simulink model "sgMdl_IO751_IO752_PROFINETMultiNode"  (R2024b)
settings: Solver=FixedStepAuto  StartTime=0.0  StopTime=inf  RelTol=1e-3  EnableMultiTasking=on
undefined symbols (not defined in the file): C, DiscIntNeverNeededParam, Ts
libraries: slrealtimeutilitieslib x80, speedgoatlib_IO752 x6, speedgoatlib_IO751 x3, simulink x2
(part 1 of 2)
Description:
  | IO751 & IO752 - PROFINET Multi-Node
settings Model: ModifiedByFormat=Speedgoat  Creator=Speedgoat  LastModifiedBy=Speedgoat
settings SolverCC: ConcurrentTasks=on  AlgebraicLoopSolver=TrustRegion  PositivePriorityOrder=on  InsertRTBMode=Never (minimum delay)
settings DataIOCC: SaveFormat=Array  SaveState=on  SignalLoggingName=logsOut
settings OptimizationCC: BlockReduction=off  BooleanDataType=off  OptimizeBlockIOStorage=off  BufferReuse=off  ReuseModelBlockBuffer=off  GlobalBufferReuse=off  ExpressionFolding=off  LocalBlockOutputs=off  InitFltsAndDblsToZero=on  OptimizeDataStoreBuffers=off  BusAssignmentInplaceUpdate=off
settings DebuggingCC: SaveWithParameterizedLinksMsg=none  UnderspecifiedInitializationDetection=Classic  MergeDetectMultiDrivingBlocksExec=none  CheckExecutionContextPreStartOutputMsg=on  SignalResolutionControl=TryResolveAllWithWarning  TasksWithSamePriorityMsg=none  UnconnectedInputMsg=warning  UnconnectedOutputMsg=warning  UnconnectedLineMsg=warning  SFUnexpectedBacktrackingDiag=warning  SFNoUnconditionalDefaultTransitionDiag=warning  SFExecutionAtInitializationDiag=none  ArithmeticOperatorsInVariantConditions=warning
settings HardwareCC: ProdBitPerLong=64  ProdLongLongMode=on  ProdHWDeviceType=Intel->x86-64 (Linux 64)
settings ModelReferenceCC: EnableRefExpFcnMdlSchedulingChecks=on  PropagateSignalLabelsOutOfModel=off
settings SFSimCC: SimUseLocalCustomCode=off  SimTargetLang=C++
settings RTWCC: Description=Speedgoat Real-Time Target Machine  SystemTargetFile=speedgoat.tlc  TemplateMakefile=slrealtime_default_tmf  RTWUseLocalCustomCode=off  Toolchain=Simulink Real-Time Toolchain  BuildConfiguration=Faster Runs  TargetLang=C++  GPUComputeCapability=3.5  DLArmComputeVersion=19.05
settings CodeAppCC: StateflowObjectComments=on
settings SimulinkRealTimeTargetCC: SubcomponentCodeInterfacePackaging=Reusable function  InstructionSetFMA=off  LogToMDFFile=off  SLRTFileLogMaxRuns=10
settings ConfigComp: CovMetricSettings=dw  CovSaveCumulativeToWorkspaceVar=on  CovSaveSingleToWorkspaceVar=on  CovExternalEMLEnable=off  CovSFcnEnable=off  CovBoundaryAbsTol=1.0e-5

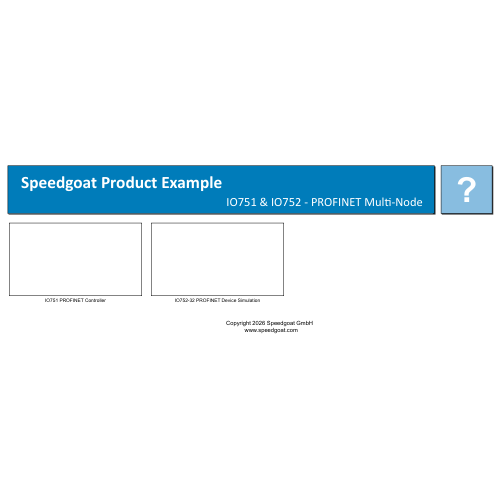
[thumbnail: Simulink's stored preview of the top-level diagram]
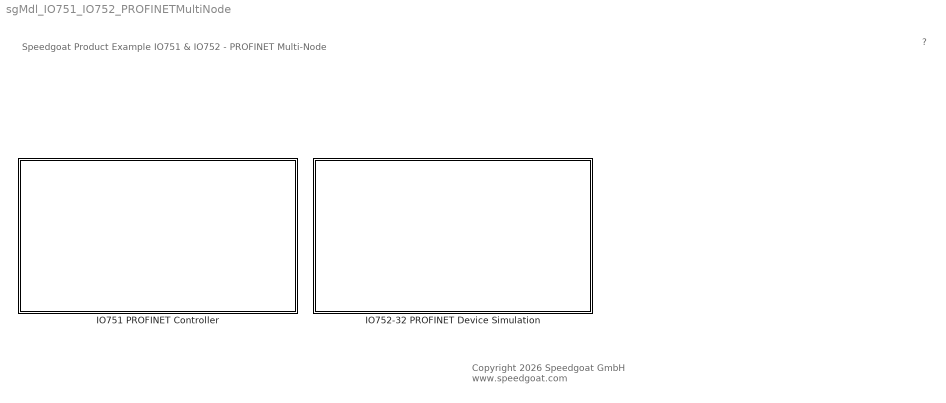
== system sgMdl_IO751_IO752_PROFINETMultiNode ==
  note: Speedgoat Product Example
      | IO751 & IO752 - PROFINET Multi-Node
  note: ?
  note: Copyright 2026 Speedgoat GmbH
      |  www.speedgoat.com
  IO751 PROFINET Controller : Subsystem
  IO752-32 PROFINET Device Simulation : Subsystem

== system sgMdl_IO751_IO752_PROFINETMultiNode/IO751 PROFINET Controller ==
  note: Send
      |
      | Send DO and AO signals to the simulated ET200SP
      | Send control signals and speed setpoints to the simulated SINAMICS drive
  note: Setup
  note: Receive
      |
      | Receive DI and AI signals from the simulated ET200SP
      | Receive status signals and actual speed values from the simulated SINAMICS drive
  "PNM Setup v2 " : speedgoatlib_IO751/PNM Setup v2   id=1  driveLetter=C:  configurationMode=Configuration file  mode=Polling mode  pciSlot=[6,0]  quantityOfAcyclicObjects=0  qtyMods=[1,0,0]  ConfigFile=which('IO751_IO752_MultiNode_m.nxd')  parOptAcyclic=off  protocol=IO751  firmware=PROFINET Controller
      settings: SourceProductName=IO751 PROFINET Controller
  Receive : Subsystem
  Send : Subsystem

== system sgMdl_IO751_IO752_PROFINETMultiNode/IO752-32 PROFINET Device Simulation ==
  Device 1 ET200SP : Subsystem
  Device 2 SINAMICS : Subsystem

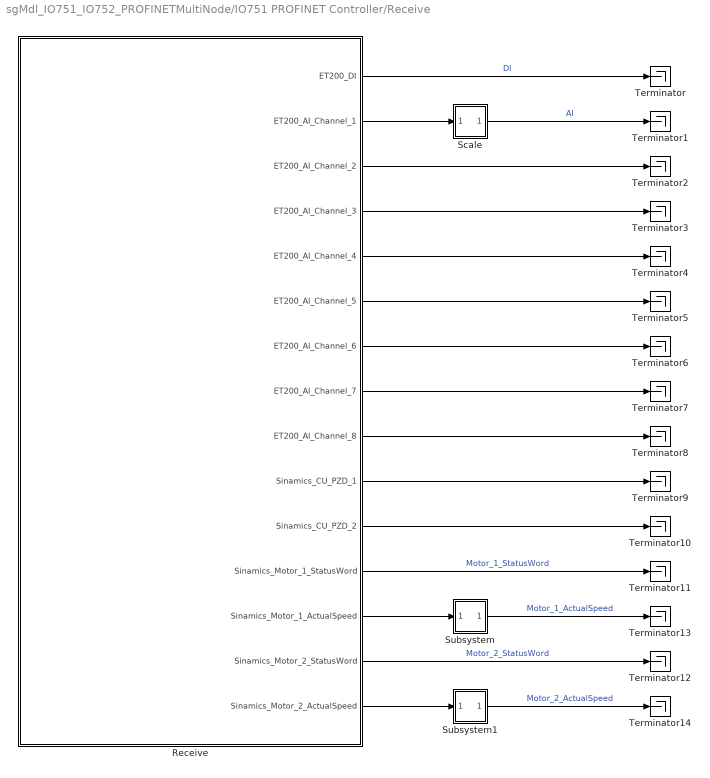
== system sgMdl_IO751_IO752_PROFINETMultiNode/IO751 PROFINET Controller/Receive ==
  Receive : Subsystem
  Scale : Subsystem
  Subsystem : Subsystem
  Subsystem1 : Subsystem
  Terminator{,1..14} (15 alike) : Terminator
  wires:
  Receive/14(Sinamics_Motor_2_StatusWord) -> Terminator12/1  "Motor_2_StatusWord"
  Receive/7(ET200_AI_Channel_6) -> Terminator6/1
  Receive/10(Sinamics_CU_PZD_1) -> Terminator9/1
  Receive/11(Sinamics_CU_PZD_2) -> Terminator10/1
  Receive/8(ET200_AI_Channel_7) -> Terminator7/1
  Receive/2(ET200_AI_Channel_1) -> Scale/1(In1)
  Receive/9(ET200_AI_Channel_8) -> Terminator8/1
  Receive/1(ET200_DI) -> Terminator/1  "DI"
  Receive/4(ET200_AI_Channel_3) -> Terminator3/1
  Receive/12(Sinamics_Motor_1_StatusWord) -> Terminator11/1  "Motor_1_StatusWord"
  Receive/3(ET200_AI_Channel_2) -> Terminator2/1
  Receive/6(ET200_AI_Channel_5) -> Terminator5/1
  Receive/5(ET200_AI_Channel_4) -> Terminator4/1
  Receive/13(Sinamics_Motor_1_ActualSpeed) -> Subsystem/1(In1)
  Subsystem/1(Out1) -> Terminator13/1  "Motor_1_ActualSpeed"
  Receive/15(Sinamics_Motor_2_ActualSpeed) -> Subsystem1/1(In1)
  Subsystem1/1(Out1) -> Terminator14/1  "Motor_2_ActualSpeed"
  Scale/1(Out1) -> Terminator1/1  "AI"

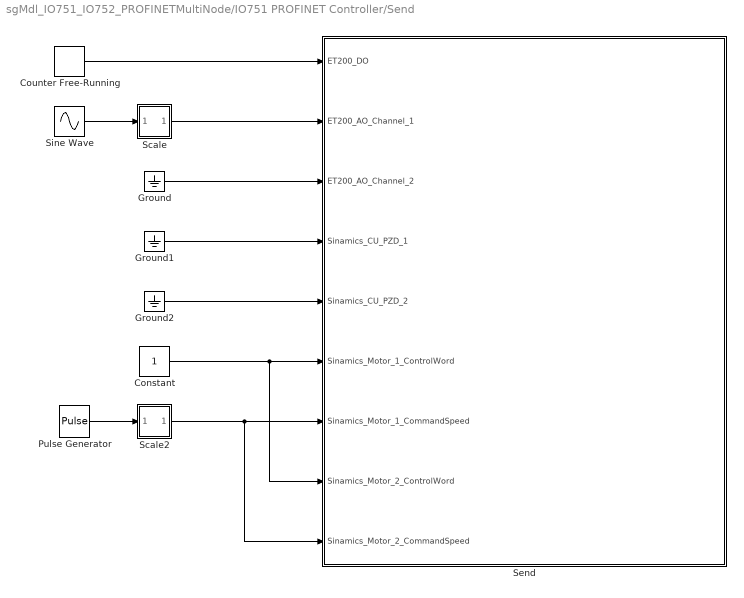
== system sgMdl_IO751_IO752_PROFINETMultiNode/IO751 PROFINET Controller/Send ==
  Constant : Constant  OutDataTypeStr=Inherit: Inherit via back propagation
  Counter Free-Running : simulink/Sources/Counter Free-Running  NumBits=16  tsamp=Ts
  Ground : Ground
  Ground1 : Ground
  Ground2 : Ground
  Pulse Generator : DiscretePulseGenerator  Amplitude=1000  Period=1/Ts*2  PulseWidth=(1/Ts*2)/2  SampleTime=Ts
  Scale : Subsystem
  Scale2 : Subsystem
  Send : Subsystem
  Sine Wave : Sin  SineType=Sample based  Amplitude=10  Frequency=180  Samples=1/Ts*4  SampleTime=Ts
  wires:
  Ground1/1 -> Send/4(Sinamics_CU_PZD_1)
  Ground/1 -> Send/3(ET200_AO_Channel_2)
  Ground2/1 -> Send/5(Sinamics_CU_PZD_2)
  Constant/1 -> Send/8(Sinamics_Motor_2_ControlWord), Send/6(Sinamics_Motor_1_ControlWord)
  Counter Free-Running/1 -> Send/1(ET200_DO)
  Sine Wave/1 -> Scale/1(In1)
  Scale/1(Out1) -> Send/2(ET200_AO_Channel_1)
  Scale2/1(Out1) -> Send/9(Sinamics_Motor_2_CommandSpeed), Send/7(Sinamics_Motor_1_CommandSpeed)
  Pulse Generator/1 -> Scale2/1(In1)

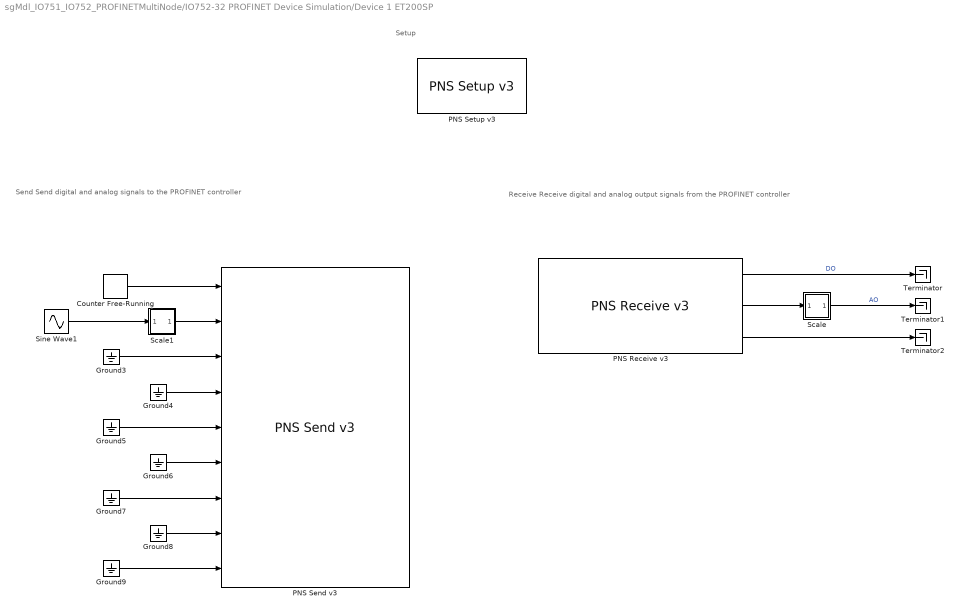
== system sgMdl_IO751_IO752_PROFINETMultiNode/IO752-32 PROFINET Device Simulation/Device 1 ET200SP ==
  note: Receive
      |
      | Receive digital and analog output signals from the PROFINET controller
  note: Setup
  note: Send
      |
      | Send digital and analog signals to the PROFINET controller
  Counter Free-Running : simulink/Sources/Counter Free-Running  NumBits=8  tsamp=Ts
  Ground{3..9} (7 alike) : Ground
  PNS Receive v3 : speedgoatlib_IO752/PNS Receive v3  id=[2 1]  SampleTime=Ts  DataLevel=Data Item  GroupDataItems=off  PortLabel1=off  PortLabel2=on  PortLabel3=off  PnModuleConfig="{ '0', '', 'IM 155-6 PN ST V4.1', '673536', '', '', 'DIM ST V4.1', '', '', '0', '1', ''; '0', '1', '  IM 155-6 PN ST V4.1', '673536', '2', '', 'DIM PN ST V4.1', '1', '', '', '', ''; '0', '32768', '  PN-IO', '673536', '32770', '', 'IDS_1I ST V4.1', '1', '', '', '', ''; '0', '32769', '  Port 1 (2xRJ45)', '673536', '49152', '', 'IDS_1P1 ST RJ45 V3.3', '0', '', '', '', ''; '0', '32770', '  Port 2 (2xRJ45)', '673536', '49152', '', 'IDS_1P2 ST RJ45 V3.3', '0', '', '', '', ''; '1', '', 'DI 8x24VDC ST V1.1', '19787', '', '', 'DI 8x24VDC ST V1.1', '0', '', '', '', ''; '1', '1', '  DI 8x24VDC ST V1.1', '19787', '8', '', 'DI 8x24VDC ST V1.1_01', '1', '{\"Inputs\",[3],[1]}', '', '', ''; '2', '', 'DQ 16x24VDC/0.5A ST V1.1', '19852', '', '', 'DQ 16x24VDC/0,5A ST V1.1', '0', '', '', '', ''; '2', '1', '  DQ 16x24VDC/0.5A ST V1.1', '19852', '16', '', 'DQ 16x24VDC/0,5A ST V1.1_01', '1', '', '{\"Outputs\",[5],[1]}', '', ''; '3', '', 'AI 8xU BA V1.0', '19022', '', '', 'AI 8xU BA', '0', '', '', '', ''; '3', '1', '  AI 8xU BA V1.0', '19022', '8', '', 'AI 8xU BA_01', '1', '{\"I-channel 0\",[4],[1];\"I-channel 1\",[4],[1];\"I-channel 2\",[4],[1];\"I-channel 3\",[4],[1];\"I-channel 4\",[4],[1];\"I-channel 5\",[4],[1];\"I-channel 6\",[4],[1];\"I-channel 7\",[4],[1]}', '', '', ''; '4', '', 'AQ 2xU ST V1.0', '19082', '', '', 'AQ 2xU ST', '0', '', '', '', ''; '4', '1', '  AQ 2xU ST V1.0', '19082', '2', '', 'AQ 2xU ST_01', '1', '', '{\"O-channel 0\",[4],[1];\"O-channel 1\",[4],[1]}', '', '' }"
      settings: SourceProductName=IO752 PROFINET Device
  PNS Send v3 : speedgoatlib_IO752/PNS Send v3  id=[2 1]  SampleTime=Ts  DataLevel=Data Item  GroupDataItems=off  PortLabel1=off  PortLabel2=on  PortLabel3=off  PnModuleConfig="{ '0', '', 'IM 155-6 PN ST V4.1', '673536', '', '', 'DIM ST V4.1', '', '', '0', '1', ''; '0', '1', '  IM 155-6 PN ST V4.1', '673536', '2', '', 'DIM PN ST V4.1', '1', '', '', '', ''; '0', '32768', '  PN-IO', '673536', '32770', '', 'IDS_1I ST V4.1', '1', '', '', '', ''; '0', '32769', '  Port 1 (2xRJ45)', '673536', '49152', '', 'IDS_1P1 ST RJ45 V3.3', '0', '', '', '', ''; '0', '32770', '  Port 2 (2xRJ45)', '673536', '49152', '', 'IDS_1P2 ST RJ45 V3.3', '0', '', '', '', ''; '1', '', 'DI 8x24VDC ST V1.1', '19787', '', '', 'DI 8x24VDC ST V1.1', '0', '', '', '', ''; '1', '1', '  DI 8x24VDC ST V1.1', '19787', '8', '', 'DI 8x24VDC ST V1.1_01', '1', '{\"Inputs\",[3],[1]}', '', '', ''; '2', '', 'DQ 16x24VDC/0.5A ST V1.1', '19852', '', '', 'DQ 16x24VDC/0,5A ST V1.1', '0', '', '', '', ''; '2', '1', '  DQ 16x24VDC/0.5A ST V1.1', '19852', '16', '', 'DQ 16x24VDC/0,5A ST V1.1_01', '1', '', '{\"Outputs\",[5],[1]}', '', ''; '3', '', 'AI 8xU BA V1.0', '19022', '', '', 'AI 8xU BA', '0', '', '', '', ''; '3', '1', '  AI 8xU BA V1.0', '19022', '8', '', 'AI 8xU BA_01', '1', '{\"I-channel 0\",[4],[1];\"I-channel 1\",[4],[1];\"I-channel 2\",[4],[1];\"I-channel 3\",[4],[1];\"I-channel 4\",[4],[1];\"I-channel 5\",[4],[1];\"I-channel 6\",[4],[1];\"I-channel 7\",[4],[1]}', '', '', ''; '4', '', 'AQ 2xU ST V1.0', '19082', '', '', 'AQ 2xU ST', '0', '', '', '', ''; '4', '1', '  AQ 2xU ST V1.0', '19082', '2', '', 'AQ 2xU ST_01', '1', '', '{\"O-channel 0\",[4],[1];\"O-channel 1\",[4],[1]}', '', '' }"
      settings: SourceProductName=IO752 PROFINET Device
  PNS Setup v3 : speedgoatlib_IO752/PNS Setup v3  id=[2 1]  PciSlot=[11,0]  StationName='et200sp'  BusStart=On model start  SystemRedundancy=off  RecordSuccess=on  GsdFile=[pwd, '\IO751_IO752_files\GSDML-V2.33-Siemens-ET200SP-20171124.xml']  VendorId=42  DeviceId=787  OptionalIdentity=off  DeviceType='cifxrepns'  OrderId='1250.1'  HwRev=2  SwRevPrefix='V'  SwRev=[3,0,0]  SerialNumber='0'  ModuleConfigTable="{ '0', '', 'IM 155-6 PN ST V4.1', '673536', '', '', 'DIM ST V4.1', '', '', '0', '1', ''; '0', '1', '  IM 155-6 PN ST V4.1', '673536', '2', '', 'DIM PN ST V4.1', '1', '', '', '', ''; '0', '32768', '  PN-IO', '673536', '32770', '', 'IDS_1I ST V4.1', '1', '', '', '', ''; '0', '32769', '  Port 1 (2xRJ45)', '673536', '49152', '', 'IDS_1P1 ST RJ45 V3.3', '0', '', '', '', ''; '0', '32770', '  Port 2 (2xRJ45)', '673536', '49152', '', 'IDS_1P2 ST RJ45 V3.3', '0', '', '', '', ''; '1', '', 'DI 8x24VDC ST V1.1', '19787', '', '', 'DI 8x24VDC ST V1.1', '0', '', '', '', ''; '1', '1', '  DI 8x24VDC ST V1.1', '19787', '8', '', 'DI 8x24VDC ST V1.1_01', '1', '{\"Inputs\",[3],[1]}', '', '', ''; '2', '', 'DQ 16x24VDC/0.5A ST V1.1', '19852', '', '', 'DQ 16x24VDC/0,5A ST V1.1', '0', '', '', '', ''; '2', '1', '  DQ 16x24VDC/0.5A ST V1.1', '19852', '16', '', 'DQ 16x24VDC/0,5A ST V1.1_01', '1', '', '{\"Outputs\",[5],[1]}', '', ''; '3', '', 'AI 8xU BA V1.0', '19022', '', '', 'AI 8xU BA', '0', '', '', '', ''; '3', '1', '  AI 8xU BA V1.0', '19022', '8', '', 'AI 8xU BA_01', '1', '{\"I-channel 0\",[4],[1];\"I-channel 1\",[4],[1];\"I-channel 2\",[4],[1];\"I-channel 3\",[4],[1];\"I-channel 4\",[4],[1];\"I-channel 5\",[4],[1];\"I-channel 6\",[4],[1];\"I-channel 7\",[4],[1]}', '', '', ''; '4', '', 'AQ 2xU ST V1.0', '19082', '', '', 'AQ 2xU ST', '0', '', '', '', ''; '4', '1', '  AQ 2xU ST V1.0', '19082', '2', '', 'AQ 2xU ST_01', '1', '', '{\"O-channel 0\",[4],[1];\"O-channel 1\",[4],[1]}', '', '' }"
      settings: SourceProductName=IO752 PROFINET Device
  Scale : Subsystem
  Scale1 : Subsystem
  Sine Wave1 : Sin  SineType=Sample based  Amplitude=5  Frequency=180  Samples=1/Ts*4  SampleTime=Ts
  Terminator : Terminator
  Terminator1 : Terminator
  Terminator2 : Terminator
  wires:
  Ground5/1 -> PNS Send v3/5
  PNS Receive v3/3 -> Terminator2/1
  Ground8/1 -> PNS Send v3/8
  Scale/1(Out1) -> Terminator1/1  "AO"
  PNS Receive v3/2 -> Scale/1(In1)
  Ground9/1 -> PNS Send v3/9
  Counter Free-Running/1 -> PNS Send v3/1
  Ground6/1 -> PNS Send v3/6
  Ground3/1 -> PNS Send v3/3
  Sine Wave1/1 -> Scale1/1(In1)
  Ground4/1 -> PNS Send v3/4
  Scale1/1(Out1) -> PNS Send v3/2
  PNS Receive v3/1 -> Terminator/1  "DO"
  Ground7/1 -> PNS Send v3/7

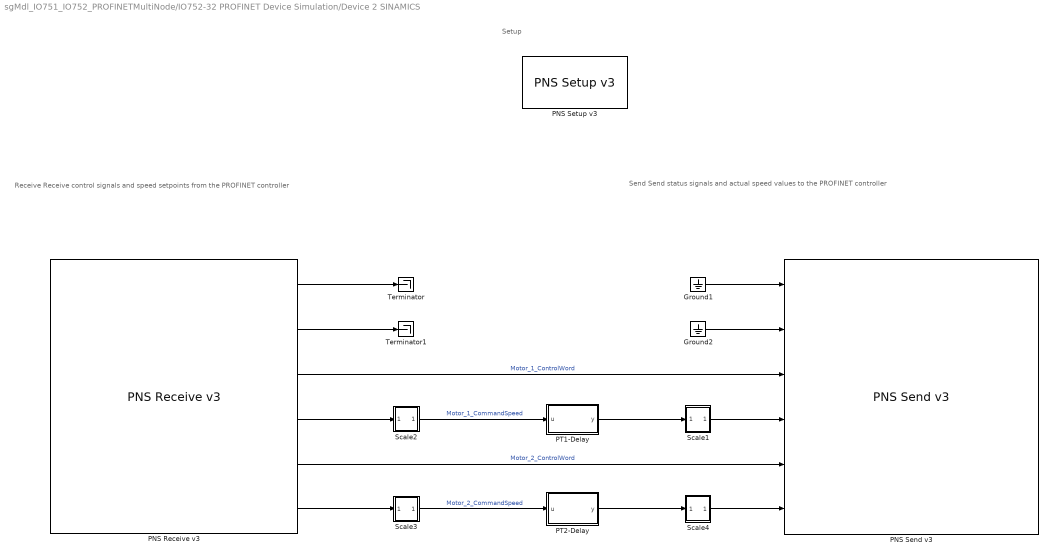
== system sgMdl_IO751_IO752_PROFINETMultiNode/IO752-32 PROFINET Device Simulation/Device 2 SINAMICS ==
  note: Send
      |
      | Send status signals and actual speed values to the PROFINET controller
  note: Setup
  note: Receive
      |
      | Receive control signals and speed setpoints from the PROFINET controller
  Ground1 : Ground
  Ground2 : Ground
  PNS Receive v3 : speedgoatlib_IO752/PNS Receive v3  id=[2 2]  SampleTime=Ts  DataLevel=Data Item  GroupDataItems=off  PortLabel1=on  PortLabel2=on  PortLabel3=off  PnModuleConfig="{ '0', '', 'SINAMICS S120/S150 CU320-2 PN V4.8', '131850', '', '', 'IDD_CU320PN-V4.8', '', '', '0', '0', ''; '0', '1', '  SINAMICS S120/S150 CU320-2 PN V4.8', '131850', '2', '', 'IDS_DAP_CU320PN-V4.8', '1', '', '', '', ''; '0', '32768', '  PN-IO', '131850', '3', '', 'IDS_IF_CU320PN-V4.8', '1', '', '', '', ''; '0', '32769', '  Port 1', '131850', '4', '', 'IDS_P1_CU320PN-V4.8', '1', '', '', '', ''; '0', '32770', '  Port 2', '131850', '5', '', 'IDS_P2_CU320PN-V4.8', '1', '', '', '', ''; '1', '', 'DO Control Unit', '805371922', '', '', 'IDM_CU_45_INT', '0', '', '', '', ''; '1', '1', '  Module Access Point', '805371922', '268500991', '14848', 'IDS_MAP1', '1', '', '', '', ''; '1', '2', '  without PROFIsafe', '805371922', '5001', '14848', 'IDS_NOSAFE', '1', '', '', '', ''; '1', '3', '  SIEMENS telegram 390, PZD-2/2', '805371922', '1342177670', '14848', 'IDS_TEL390_INT2', '0', '{\"Status word or actual value\",[5],[1];\"Status word or actual value\",[5],[1]}', '{\"Control word or setpoint\",[5],[1];\"Control word or setpoint\",[5],[1]}', '', ''; '2', '', 'DO SERVO', '805372083', '', '', 'IDM_SERVO_46_INT', '0', '', '', '', ''; '2', '1', '  Module Access Point', '805372083', '65535', '14848', 'IDS_MAP', '1', '', '', '', ''; '2', '2', '  empty submodule', '805372083', '5000', '14848', 'IDS_EMPTY', '0', '', '', '', ''; '2', '3', '  Standard telegram 1, PZD-2/2', '805372083', '1', '14848', 'IDS_TEL1', '0', '{\"Status word or actual value\",[5],[1];\"Status word or actual value\",[5],[1]}', '{\"Control word or setpoint\",[5],[1];\"Control word or setpoint\",[5],[1]}', '', ''; '3', '', 'DO SERVO', '805372083', '', '', 'IDM_SERVO_46_INT', '0', '', '', '', ''; '3', '1', '  Module Access Point', '805372083', '65535', '14848', 'IDS_MAP', '1', '', '', '', ''; '3', '2', '  empty submodule', '805372083', '5000', '14848', 'IDS_EMPTY', '0', '', '', '', ''; '3', '3', '  Standard telegram 1, PZD-2/2', '805372083', '1', '14848', 'IDS_TEL1', '0', '{\"Status word or actual value\",[5],[1];\"Status word or actual value\",[5],[1]}', '{\"Control word or setpoint\",[5],[1];\"Control word or setpoint\",[5],[1]}', '', '' }"
      settings: SourceProductName=IO752 PROFINET Device
  PNS Send v3 : speedgoatlib_IO752/PNS Send v3  id=[2 2]  SampleTime=Ts  DataLevel=Data Item  GroupDataItems=off  PortLabel1=on  PortLabel2=on  PortLabel3=off  PnModuleConfig="{ '0', '', 'SINAMICS S120/S150 CU320-2 PN V4.8', '131850', '', '', 'IDD_CU320PN-V4.8', '', '', '0', '0', ''; '0', '1', '  SINAMICS S120/S150 CU320-2 PN V4.8', '131850', '2', '', 'IDS_DAP_CU320PN-V4.8', '1', '', '', '', ''; '0', '32768', '  PN-IO', '131850', '3', '', 'IDS_IF_CU320PN-V4.8', '1', '', '', '', ''; '0', '32769', '  Port 1', '131850', '4', '', 'IDS_P1_CU320PN-V4.8', '1', '', '', '', ''; '0', '32770', '  Port 2', '131850', '5', '', 'IDS_P2_CU320PN-V4.8', '1', '', '', '', ''; '1', '', 'DO Control Unit', '805371922', '', '', 'IDM_CU_45_INT', '0', '', '', '', ''; '1', '1', '  Module Access Point', '805371922', '268500991', '14848', 'IDS_MAP1', '1', '', '', '', ''; '1', '2', '  without PROFIsafe', '805371922', '5001', '14848', 'IDS_NOSAFE', '1', '', '', '', ''; '1', '3', '  SIEMENS telegram 390, PZD-2/2', '805371922', '1342177670', '14848', 'IDS_TEL390_INT2', '0', '{\"Status word or actual value\",[5],[1];\"Status word or actual value\",[5],[1]}', '{\"Control word or setpoint\",[5],[1];\"Control word or setpoint\",[5],[1]}', '', ''; '2', '', 'DO SERVO', '805372083', '', '', 'IDM_SERVO_46_INT', '0', '', '', '', ''; '2', '1', '  Module Access Point', '805372083', '65535', '14848', 'IDS_MAP', '1', '', '', '', ''; '2', '2', '  empty submodule', '805372083', '5000', '14848', 'IDS_EMPTY', '0', '', '', '', ''; '2', '3', '  Standard telegram 1, PZD-2/2', '805372083', '1', '14848', 'IDS_TEL1', '0', '{\"Status word or actual value\",[5],[1];\"Status word or actual value\",[5],[1]}', '{\"Control word or setpoint\",[5],[1];\"Control word or setpoint\",[5],[1]}', '', ''; '3', '', 'DO SERVO', '805372083', '', '', 'IDM_SERVO_46_INT', '0', '', '', '', ''; '3', '1', '  Module Access Point', '805372083', '65535', '14848', 'IDS_MAP', '1', '', '', '', ''; '3', '2', '  empty submodule', '805372083', '5000', '14848', 'IDS_EMPTY', '0', '', '', '', ''; '3', '3', '  Standard telegram 1, PZD-2/2', '805372083', '1', '14848', 'IDS_TEL1', '0', '{\"Status word or actual value\",[5],[1];\"Status word or actual value\",[5],[1]}', '{\"Control word or setpoint\",[5],[1];\"Control word or setpoint\",[5],[1]}', '', '' }"
      settings: SourceProductName=IO752 PROFINET Device
  PNS Setup v3 : speedgoatlib_IO752/PNS Setup v3  id=[2 2]  PciSlot=[11,0]  StationName='sinamics-s120-cu320-2pn'  BusStart=On model start  SystemRedundancy=off  RecordSuccess=on  GsdFile=[pwd, '\IO751_IO752_files\GSDML-V2.32-Siemens-Sinamics_S_CU3x0-20160531.xml']  VendorId=42  DeviceId=1281  OptionalIdentity=off  DeviceType='cifxrepns'  OrderId='1250.1'  HwRev=2  SwRevPrefix='V'  SwRev=[3,0,0]  SerialNumber='0'  ModuleConfigTable="{ '0', '', 'SINAMICS S120/S150 CU320-2 PN V4.8', '131850', '', '', 'IDD_CU320PN-V4.8', '', '', '0', '0', ''; '0', '1', '  SINAMICS S120/S150 CU320-2 PN V4.8', '131850', '2', '', 'IDS_DAP_CU320PN-V4.8', '1', '', '', '', ''; '0', '32768', '  PN-IO', '131850', '3', '', 'IDS_IF_CU320PN-V4.8', '1', '', '', '', ''; '0', '32769', '  Port 1', '131850', '4', '', 'IDS_P1_CU320PN-V4.8', '1', '', '', '', ''; '0', '32770', '  Port 2', '131850', '5', '', 'IDS_P2_CU320PN-V4.8', '1', '', '', '', ''; '1', '', 'DO Control Unit', '805371922', '', '', 'IDM_CU_45_INT', '0', '', '', '', ''; '1', '1', '  Module Access Point', '805371922', '268500991', '14848', 'IDS_MAP1', '1', '', '', '', ''; '1', '2', '  without PROFIsafe', '805371922', '5001', '14848', 'IDS_NOSAFE', '1', '', '', '', ''; '1', '3', '  SIEMENS telegram 390, PZD-2/2', '805371922', '1342177670', '14848', 'IDS_TEL390_INT2', '0', '{\"Status word or actual value\",[5],[1];\"Status word or actual value\",[5],[1]}', '{\"Control word or setpoint\",[5],[1];\"Control word or setpoint\",[5],[1]}', '', ''; '2', '', 'DO SERVO', '805372083', '', '', 'IDM_SERVO_46_INT', '0', '', '', '', ''; '2', '1', '  Module Access Point', '805372083', '65535', '14848', 'IDS_MAP', '1', '', '', '', ''; '2', '2', '  empty submodule', '805372083', '5000', '14848', 'IDS_EMPTY', '0', '', '', '', ''; '2', '3', '  Standard telegram 1, PZD-2/2', '805372083', '1', '14848', 'IDS_TEL1', '0', '{\"Status word or actual value\",[5],[1];\"Status word or actual value\",[5],[1]}', '{\"Control word or setpoint\",[5],[1];\"Control word or setpoint\",[5],[1]}', '', ''; '3', '', 'DO SERVO', '805372083', '', '', 'IDM_SERVO_46_INT', '0', '', '', '', ''; '3', '1', '  Module Access Point', '805372083', '65535', '14848', 'IDS_MAP', '1', '', '', '', ''; '3', '2', '  empty submodule', '805372083', '5000', '14848', 'IDS_EMPTY', '0', '', '', '', ''; '3', '3', '  Standard telegram 1, PZD-2/2', '805372083', '1', '14848', 'IDS_TEL1', '0', '{\"Status word or actual value\",[5],[1];\"Status word or actual value\",[5],[1]}', '{\"Control word or setpoint\",[5],[1];\"Control word or setpoint\",[5],[1]}', '', '' }"
      settings: SourceProductName=IO752 PROFINET Device
  PT1-Delay : Subsystem
  PT2-Delay : Subsystem
  Scale1 : Subsystem
  Scale2 : Subsystem
  Scale3 : Subsystem
  Scale4 : Subsystem
  Terminator : Terminator
  Terminator1 : Terminator
  wires:
  PNS Receive v3/1 -> Terminator/1
  PNS Receive v3/2 -> Terminator1/1
  PNS Receive v3/4 -> Scale2/1(In1)
  PNS Receive v3/6 -> Scale3/1(In1)
  Scale3/1(Out1) -> PT2-Delay/1(u)  "Motor_2_CommandSpeed"
  PT2-Delay/1(y) -> Scale4/1(In2)
  PT1-Delay/1(y) -> Scale1/1(In2)
  Scale2/1(Out1) -> PT1-Delay/1(u)  "Motor_1_CommandSpeed"
  Scale1/1(Out1) -> PNS Send v3/4
  Scale4/1(Out1) -> PNS Send v3/6
  PNS Receive v3/5 -> PNS Send v3/5  "Motor_2_ControlWord"
  PNS Receive v3/3 -> PNS Send v3/3  "Motor_1_ControlWord"
  Ground1/1 -> PNS Send v3/1
  Ground2/1 -> PNS Send v3/2

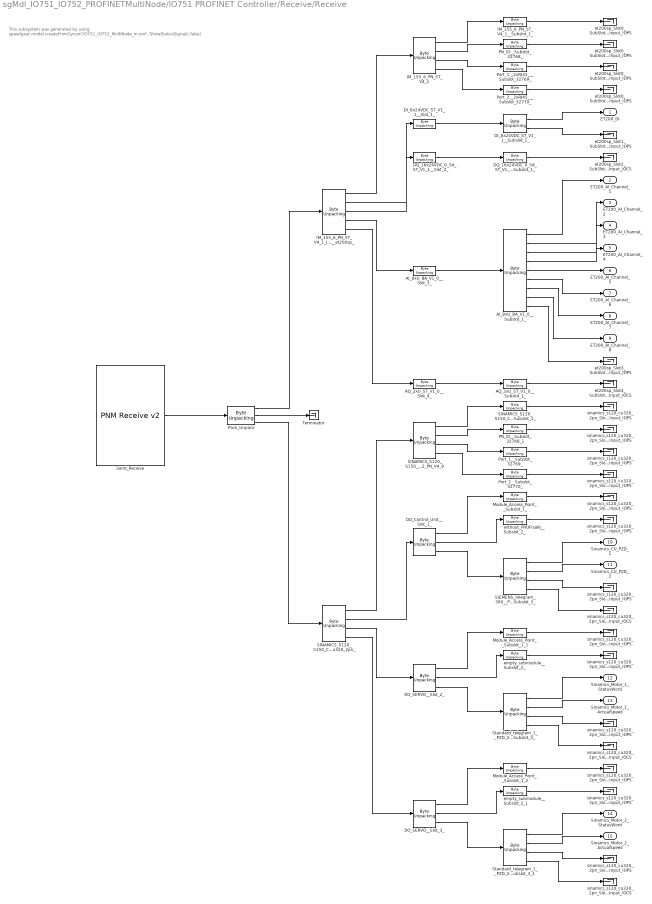
== system sgMdl_IO751_IO752_PROFINETMultiNode/IO751 PROFINET Controller/Receive/Receive ==
  note: This subsystem was generated by using speedgoat.model.createFromSycon('IO751_IO752_MultiNode_m.xml','ShowStatusSignals',false)
  AI_8xU_BA_V1_0__Slot_3_ : slrealtimeutilitieslib/Byte Unpacking  MaskUnpackedDataTypes={'uint8'}  MaskUnpackedDataSizes={[17]}  MaskAlignment=1
  AI_8xU_BA_V1_0__Subslot_1_ : slrealtimeutilitieslib/Byte Unpacking  MaskUnpackedDataTypes={'int16','int16','int16','int16','int16','int16','int16','int16','uint8'}  MaskUnpackedDataSizes={[1],[1],[1],[1],[1],[1],[1],[1],[1]}  MaskAlignment=1
  AQ_2xU_ST_V1_0__Slot_4_ : slrealtimeutilitieslib/Byte Unpacking  MaskUnpackedDataTypes={'uint8'}  MaskUnpackedDataSizes={[1]}  MaskAlignment=1
  AQ_2xU_ST_V1_0__Subslot_1_ : slrealtimeutilitieslib/Byte Unpacking  MaskUnpackedDataTypes={'uint8'}  MaskUnpackedDataSizes={[1]}  MaskAlignment=1
  DI_8x24VDC_ST_V1_1__Slot_1_ : slrealtimeutilitieslib/Byte Unpacking  MaskUnpackedDataTypes={'uint8'}  MaskUnpackedDataSizes={[2]}  MaskAlignment=1
  DI_8x24VDC_ST_V1_1__Subslot_1_ : slrealtimeutilitieslib/Byte Unpacking  MaskUnpackedDataTypes={'uint8','uint8'}  MaskUnpackedDataSizes={[1],[1]}  MaskAlignment=1
  DO_Control_Unit__Slot_1_ : slrealtimeutilitieslib/Byte Unpacking  MaskUnpackedDataTypes={'uint8','uint8','uint8'}  MaskUnpackedDataSizes={[1],[1],[6]}  MaskAlignment=1
  DO_SERVO__Slot_2_ : slrealtimeutilitieslib/Byte Unpacking  MaskUnpackedDataTypes={'uint8','uint8','uint8'}  MaskUnpackedDataSizes={[1],[1],[6]}  MaskAlignment=1
  DO_SERVO__Slot_3_ : slrealtimeutilitieslib/Byte Unpacking  MaskUnpackedDataTypes={'uint8','uint8','uint8'}  MaskUnpackedDataSizes={[1],[1],[6]}  MaskAlignment=1
  DQ_16x24VDC_0_5A_ST_V1_1__Slot_2_ : slrealtimeutilitieslib/Byte Unpacking  MaskUnpackedDataTypes={'uint8'}  MaskUnpackedDataSizes={[1]}  MaskAlignment=1
  DQ_16x24VDC_0_5A_ST_V1_1__Subslot_1_ : slrealtimeutilitieslib/Byte Unpacking  MaskUnpackedDataTypes={'uint8'}  MaskUnpackedDataSizes={[1]}  MaskAlignment=1
  IM_155_6_PN_ST_V4_1 : slrealtimeutilitieslib/Byte Unpacking  MaskUnpackedDataTypes={'uint8','uint8','uint8','uint8'}  MaskUnpackedDataSizes={[1],[1],[1],[1]}  MaskAlignment=1
  IM_155_6_PN_ST_V4_1_IM_155_6_PN_ST_V4_1__et200sp_ : slrealtimeutilitieslib/Byte Unpacking  MaskUnpackedDataTypes={'uint8','uint8','uint8','uint8','uint8'}  MaskUnpackedDataSizes={[4],[2],[1],[17],[1]}  MaskAlignment=1
  IM_155_6_PN_ST_V4_1__Subslot_1_ : slrealtimeutilitieslib/Byte Unpacking  MaskUnpackedDataTypes={'uint8'}  MaskUnpackedDataSizes={[1]}  MaskAlignment=1
  Module_Access_Point__Subslot_1_ : slrealtimeutilitieslib/Byte Unpacking  MaskUnpackedDataTypes={'uint8'}  MaskUnpackedDataSizes={[1]}  MaskAlignment=1
  Module_Access_Point__Subslot_1_1 : slrealtimeutilitieslib/Byte Unpacking  MaskUnpackedDataTypes={'uint8'}  MaskUnpackedDataSizes={[1]}  MaskAlignment=1
  Module_Access_Point__Subslot_1_2 : slrealtimeutilitieslib/Byte Unpacking  MaskUnpackedDataTypes={'uint8'}  MaskUnpackedDataSizes={[1]}  MaskAlignment=1
  PN_IO__Subslot_32768_ : slrealtimeutilitieslib/Byte Unpacking  MaskUnpackedDataTypes={'uint8'}  MaskUnpackedDataSizes={[1]}  MaskAlignment=1
  PN_IO__Subslot_32768_1 : slrealtimeutilitieslib/Byte Unpacking  MaskUnpackedDataTypes={'uint8'}  MaskUnpackedDataSizes={[1]}  MaskAlignment=1
  Pack_Unpack : slrealtimeutilitieslib/Byte Unpacking  MaskUnpackedDataTypes={'uint8','uint8','uint8'}  MaskUnpackedDataSizes={[25],[3],[28]}  MaskAlignment=1
  Port_1__2xRJ45___Subslot_32769_ : slrealtimeutilitieslib/Byte Unpacking  MaskUnpackedDataTypes={'uint8'}  MaskUnpackedDataSizes={[1]}  MaskAlignment=1
  Port_1__Subslot_32769_ : slrealtimeutilitieslib/Byte Unpacking  MaskUnpackedDataTypes={'uint8'}  MaskUnpackedDataSizes={[1]}  MaskAlignment=1
  Port_2__2xRJ45___Subslot_32770_ : slrealtimeutilitieslib/Byte Unpacking  MaskUnpackedDataTypes={'uint8'}  MaskUnpackedDataSizes={[1]}  MaskAlignment=1
  Port_2__Subslot_32770_ : slrealtimeutilitieslib/Byte Unpacking  MaskUnpackedDataTypes={'uint8'}  MaskUnpackedDataSizes={[1]}  MaskAlignment=1
  SIEMENS_telegram_390__PZD_2_2__Subslot_3_ : slrealtimeutilitieslib/Byte Unpacking  MaskUnpackedDataTypes={'uint16','uint16','uint8','uint8'}  MaskUnpackedDataSizes={[1],[1],[1],[1]}  MaskAlignment=1
  SINAMICS_S120_S150_CU320_2_PN_V4_8 : slrealtimeutilitieslib/Byte Unpacking  MaskUnpackedDataTypes={'uint8','uint8','uint8','uint8'}  MaskUnpackedDataSizes={[1],[1],[1],[1]}  MaskAlignment=1
  SINAMICS_S120_S150_CU320_2_PN_V4_8_SINAMICS_S120_S150_CU320_2_PN_V4_8__sinamics_s120_cu320_2pn_ : slrealtimeutilitieslib/Byte Unpacking  MaskUnpackedDataTypes={'uint8','uint8','uint8','uint8'}  MaskUnpackedDataSizes={[4],[8],[8],[8]}  MaskAlignment=1
  SINAMICS_S120_S150_CU320_2_PN_V4_8__Subslot_1_ : slrealtimeutilitieslib/Byte Unpacking  MaskUnpackedDataTypes={'uint8'}  MaskUnpackedDataSizes={[1]}  MaskAlignment=1
  Send_Receive : speedgoatlib_IO751/PNM Receive v2   id=1  portType=1 port with n element vector of type UINT8  inputOutput=56  sampleTime=Ts
      settings: SourceProductName=IO751 PROFINET Controller
  Standard_telegram_1__PZD_2_2__Subslot_3_ : slrealtimeutilitieslib/Byte Unpacking  MaskUnpackedDataTypes={'uint16','int16','uint8','uint8'}  MaskUnpackedDataSizes={[1],[1],[1],[1]}  MaskAlignment=1
  Standard_telegram_1__PZD_2_2__Subslot_3_1 : slrealtimeutilitieslib/Byte Unpacking  MaskUnpackedDataTypes={'uint16','int16','uint8','uint8'}  MaskUnpackedDataSizes={[1],[1],[1],[1]}  MaskAlignment=1
  Terminator : Terminator
  empty_submodule__Subslot_2_ : slrealtimeutilitieslib/Byte Unpacking  MaskUnpackedDataTypes={'uint8'}  MaskUnpackedDataSizes={[1]}  MaskAlignment=1
  empty_submodule__Subslot_2_1 : slrealtimeutilitieslib/Byte Unpacking  MaskUnpackedDataTypes={'uint8'}  MaskUnpackedDataSizes={[1]}  MaskAlignment=1
  et200sp_Slot0_SubSlot1_Input_IOPS : Terminator
  et200sp_Slot0_SubSlot32768_Input_IOPS : Terminator
  et200sp_Slot0_SubSlot32769_Input_IOPS : Terminator
  et200sp_Slot0_SubSlot32770_Input_IOPS : Terminator
  et200sp_Slot1_SubSlot1_Input_IOPS : Terminator
  et200sp_Slot2_SubSlot1_Input_IOCS : Terminator
  et200sp_Slot3_SubSlot1_Input_IOPS : Terminator
  et200sp_Slot4_SubSlot1_Input_IOCS : Terminator
  sinamics_s120_cu320_2pn_Slot0_SubSlot1_Input_IOPS : Terminator
  sinamics_s120_cu320_2pn_Slot0_SubSlot32768_Input_IOPS : Terminator
  sinamics_s120_cu320_2pn_Slot0_SubSlot32769_Input_IOPS : Terminator
  sinamics_s120_cu320_2pn_Slot0_SubSlot32770_Input_IOPS : Terminator
  sinamics_s120_cu320_2pn_Slot1_SubSlot1_Input_IOPS : Terminator
  sinamics_s120_cu320_2pn_Slot1_SubSlot2_Input_IOPS : Terminator
  sinamics_s120_cu320_2pn_Slot1_SubSlot3_Input_IOCS : Terminator
  sinamics_s120_cu320_2pn_Slot1_SubSlot3_Input_IOPS : Terminator
  sinamics_s120_cu320_2pn_Slot2_SubSlot1_Input_IOPS : Terminator
  sinamics_s120_cu320_2pn_Slot2_SubSlot2_Input_IOPS : Terminator
  sinamics_s120_cu320_2pn_Slot2_SubSlot3_Input_IOCS : Terminator
  sinamics_s120_cu320_2pn_Slot2_SubSlot3_Input_IOPS : Terminator
  sinamics_s120_cu320_2pn_Slot3_SubSlot1_Input_IOPS : Terminator
  sinamics_s120_cu320_2pn_Slot3_SubSlot2_Input_IOPS : Terminator
  sinamics_s120_cu320_2pn_Slot3_SubSlot3_Input_IOCS : Terminator
  sinamics_s120_cu320_2pn_Slot3_SubSlot3_Input_IOPS : Terminator
  without_PROFIsafe__Subslot_2_ : slrealtimeutilitieslib/Byte Unpacking  MaskUnpackedDataTypes={'uint8'}  MaskUnpackedDataSizes={[1]}  MaskAlignment=1
  ET200_DI : Outport  OutDataTypeStr=uint8  PortDimensions=1
  ET200_AI_Channel_1 : Outport  Port=2  OutDataTypeStr=int16  PortDimensions=1
  ET200_AI_Channel_2 : Outport  Port=3  OutDataTypeStr=int16  PortDimensions=1
  ET200_AI_Channel_3 : Outport  Port=4  OutDataTypeStr=int16  PortDimensions=1
  ET200_AI_Channel_4 : Outport  Port=5  OutDataTypeStr=int16  PortDimensions=1
  ET200_AI_Channel_5 : Outport  Port=6  OutDataTypeStr=int16  PortDimensions=1
  ET200_AI_Channel_6 : Outport  Port=7  OutDataTypeStr=int16  PortDimensions=1
  ET200_AI_Channel_7 : Outport  Port=8  OutDataTypeStr=int16  PortDimensions=1
  ET200_AI_Channel_8 : Outport  Port=9  OutDataTypeStr=int16  PortDimensions=1
  Sinamics_CU_PZD_1 : Outport  Port=10  OutDataTypeStr=uint16  PortDimensions=1
  Sinamics_CU_PZD_2 : Outport  Port=11  OutDataTypeStr=uint16  PortDimensions=1
  Sinamics_Motor_1_StatusWord : Outport  Port=12  OutDataTypeStr=uint16  PortDimensions=1
  Sinamics_Motor_1_ActualSpeed : Outport  Port=13  OutDataTypeStr=int16  PortDimensions=1
  Sinamics_Motor_2_StatusWord : Outport  Port=14  OutDataTypeStr=uint16  PortDimensions=1
  Sinamics_Motor_2_ActualSpeed : Outport  Port=15  OutDataTypeStr=int16  PortDimensions=1
  wires:
  IM_155_6_PN_ST_V4_1__Subslot_1_/1 -> et200sp_Slot0_SubSlot1_Input_IOPS/1
  PN_IO__Subslot_32768_/1 -> et200sp_Slot0_SubSlot32768_Input_IOPS/1
  Port_1__2xRJ45___Subslot_32769_/1 -> et200sp_Slot0_SubSlot32769_Input_IOPS/1
  Port_2__2xRJ45___Subslot_32770_/1 -> et200sp_Slot0_SubSlot32770_Input_IOPS/1
  IM_155_6_PN_ST_V4_1/1 -> IM_155_6_PN_ST_V4_1__Subslot_1_/1
  IM_155_6_PN_ST_V4_1/2 -> PN_IO__Subslot_32768_/1
  IM_155_6_PN_ST_V4_1/3 -> Port_1__2xRJ45___Subslot_32769_/1
  IM_155_6_PN_ST_V4_1/4 -> Port_2__2xRJ45___Subslot_32770_/1
  DI_8x24VDC_ST_V1_1__Subslot_1_/1 -> ET200_DI/1
  DI_8x24VDC_ST_V1_1__Subslot_1_/2 -> et200sp_Slot1_SubSlot1_Input_IOPS/1
  DI_8x24VDC_ST_V1_1__Slot_1_/1 -> DI_8x24VDC_ST_V1_1__Subslot_1_/1
  DQ_16x24VDC_0_5A_ST_V1_1__Subslot_1_/1 -> et200sp_Slot2_SubSlot1_Input_IOCS/1
  DQ_16x24VDC_0_5A_ST_V1_1__Slot_2_/1 -> DQ_16x24VDC_0_5A_ST_V1_1__Subslot_1_/1
  AI_8xU_BA_V1_0__Subslot_1_/1 -> ET200_AI_Channel_1/1
  AI_8xU_BA_V1_0__Subslot_1_/2 -> ET200_AI_Channel_2/1
  AI_8xU_BA_V1_0__Subslot_1_/3 -> ET200_AI_Channel_3/1
  AI_8xU_BA_V1_0__Subslot_1_/4 -> ET200_AI_Channel_4/1
  AI_8xU_BA_V1_0__Subslot_1_/5 -> ET200_AI_Channel_5/1
  AI_8xU_BA_V1_0__Subslot_1_/6 -> ET200_AI_Channel_6/1
  AI_8xU_BA_V1_0__Subslot_1_/7 -> ET200_AI_Channel_7/1
  AI_8xU_BA_V1_0__Subslot_1_/8 -> ET200_AI_Channel_8/1
  AI_8xU_BA_V1_0__Subslot_1_/9 -> et200sp_Slot3_SubSlot1_Input_IOPS/1
  AI_8xU_BA_V1_0__Slot_3_/1 -> AI_8xU_BA_V1_0__Subslot_1_/1
  AQ_2xU_ST_V1_0__Subslot_1_/1 -> et200sp_Slot4_SubSlot1_Input_IOCS/1
  AQ_2xU_ST_V1_0__Slot_4_/1 -> AQ_2xU_ST_V1_0__Subslot_1_/1
  IM_155_6_PN_ST_V4_1_IM_155_6_PN_ST_V4_1__et200sp_/1 -> IM_155_6_PN_ST_V4_1/1
  IM_155_6_PN_ST_V4_1_IM_155_6_PN_ST_V4_1__et200sp_/2 -> DI_8x24VDC_ST_V1_1__Slot_1_/1
  IM_155_6_PN_ST_V4_1_IM_155_6_PN_ST_V4_1__et200sp_/3 -> DQ_16x24VDC_0_5A_ST_V1_1__Slot_2_/1
  IM_155_6_PN_ST_V4_1_IM_155_6_PN_ST_V4_1__et200sp_/4 -> AI_8xU_BA_V1_0__Slot_3_/1
  IM_155_6_PN_ST_V4_1_IM_155_6_PN_ST_V4_1__et200sp_/5 -> AQ_2xU_ST_V1_0__Slot_4_/1
  SINAMICS_S120_S150_CU320_2_PN_V4_8__Subslot_1_/1 -> sinamics_s120_cu320_2pn_Slot0_SubSlot1_Input_IOPS/1
  PN_IO__Subslot_32768_1/1 -> sinamics_s120_cu320_2pn_Slot0_SubSlot32768_Input_IOPS/1
  Port_1__Subslot_32769_/1 -> sinamics_s120_cu320_2pn_Slot0_SubSlot32769_Input_IOPS/1
  Port_2__Subslot_32770_/1 -> sinamics_s120_cu320_2pn_Slot0_SubSlot32770_Input_IOPS/1
  SINAMICS_S120_S150_CU320_2_PN_V4_8/1 -> SINAMICS_S120_S150_CU320_2_PN_V4_8__Subslot_1_/1
  SINAMICS_S120_S150_CU320_2_PN_V4_8/2 -> PN_IO__Subslot_32768_1/1
  SINAMICS_S120_S150_CU320_2_PN_V4_8/3 -> Port_1__Subslot_32769_/1
  SINAMICS_S120_S150_CU320_2_PN_V4_8/4 -> Port_2__Subslot_32770_/1
  Module_Access_Point__Subslot_1_/1 -> sinamics_s120_cu320_2pn_Slot1_SubSlot1_Input_IOPS/1
  without_PROFIsafe__Subslot_2_/1 -> sinamics_s120_cu320_2pn_Slot1_SubSlot2_Input_IOPS/1
  SIEMENS_telegram_390__PZD_2_2__Subslot_3_/1 -> Sinamics_CU_PZD_1/1
  SIEMENS_telegram_390__PZD_2_2__Subslot_3_/2 -> Sinamics_CU_PZD_2/1
  SIEMENS_telegram_390__PZD_2_2__Subslot_3_/3 -> sinamics_s120_cu320_2pn_Slot1_SubSlot3_Input_IOPS/1
  SIEMENS_telegram_390__PZD_2_2__Subslot_3_/4 -> sinamics_s120_cu320_2pn_Slot1_SubSlot3_Input_IOCS/1
  DO_Control_Unit__Slot_1_/1 -> Module_Access_Point__Subslot_1_/1
  DO_Control_Unit__Slot_1_/2 -> without_PROFIsafe__Subslot_2_/1
  DO_Control_Unit__Slot_1_/3 -> SIEMENS_telegram_390__PZD_2_2__Subslot_3_/1
  Module_Access_Point__Subslot_1_1/1 -> sinamics_s120_cu320_2pn_Slot2_SubSlot1_Input_IOPS/1
  empty_submodule__Subslot_2_/1 -> sinamics_s120_cu320_2pn_Slot2_SubSlot2_Input_IOPS/1
  Standard_telegram_1__PZD_2_2__Subslot_3_/1 -> Sinamics_Motor_1_StatusWord/1
  Standard_telegram_1__PZD_2_2__Subslot_3_/2 -> Sinamics_Motor_1_ActualSpeed/1
  Standard_telegram_1__PZD_2_2__Subslot_3_/3 -> sinamics_s120_cu320_2pn_Slot2_SubSlot3_Input_IOPS/1
  Standard_telegram_1__PZD_2_2__Subslot_3_/4 -> sinamics_s120_cu320_2pn_Slot2_SubSlot3_Input_IOCS/1
  DO_SERVO__Slot_2_/1 -> Module_Access_Point__Subslot_1_1/1
  DO_SERVO__Slot_2_/2 -> empty_submodule__Subslot_2_/1
  DO_SERVO__Slot_2_/3 -> Standard_telegram_1__PZD_2_2__Subslot_3_/1
  Module_Access_Point__Subslot_1_2/1 -> sinamics_s120_cu320_2pn_Slot3_SubSlot1_Input_IOPS/1
  empty_submodule__Subslot_2_1/1 -> sinamics_s120_cu320_2pn_Slot3_SubSlot2_Input_IOPS/1
  Standard_telegram_1__PZD_2_2__Subslot_3_1/1 -> Sinamics_Motor_2_StatusWord/1
  Standard_telegram_1__PZD_2_2__Subslot_3_1/2 -> Sinamics_Motor_2_ActualSpeed/1
  Standard_telegram_1__PZD_2_2__Subslot_3_1/3 -> sinamics_s120_cu320_2pn_Slot3_SubSlot3_Input_IOPS/1
  Standard_telegram_1__PZD_2_2__Subslot_3_1/4 -> sinamics_s120_cu320_2pn_Slot3_SubSlot3_Input_IOCS/1
  DO_SERVO__Slot_3_/1 -> Module_Access_Point__Subslot_1_2/1
  DO_SERVO__Slot_3_/2 -> empty_submodule__Subslot_2_1/1
  DO_SERVO__Slot_3_/3 -> Standard_telegram_1__PZD_2_2__Subslot_3_1/1
  SINAMICS_S120_S150_CU320_2_PN_V4_8_SINAMICS_S120_S150_CU320_2_PN_V4_8__sinamics_s120_cu320_2pn_/1 -> SINAMICS_S120_S150_CU320_2_PN_V4_8/1
  SINAMICS_S120_S150_CU320_2_PN_V4_8_SINAMICS_S120_S150_CU320_2_PN_V4_8__sinamics_s120_cu320_2pn_/2 -> DO_Control_Unit__Slot_1_/1
  SINAMICS_S120_S150_CU320_2_PN_V4_8_SINAMICS_S120_S150_CU320_2_PN_V4_8__sinamics_s120_cu320_2pn_/3 -> DO_SERVO__Slot_2_/1
  SINAMICS_S120_S150_CU320_2_PN_V4_8_SINAMICS_S120_S150_CU320_2_PN_V4_8__sinamics_s120_cu320_2pn_/4 -> DO_SERVO__Slot_3_/1
  Pack_Unpack/1 -> IM_155_6_PN_ST_V4_1_IM_155_6_PN_ST_V4_1__et200sp_/1
  Send_Receive/1 -> Pack_Unpack/1
  Pack_Unpack/3 -> SINAMICS_S120_S150_CU320_2_PN_V4_8_SINAMICS_S120_S150_CU320_2_PN_V4_8__sinamics_s120_cu320_2pn_/1
  Pack_Unpack/2 -> Terminator/1

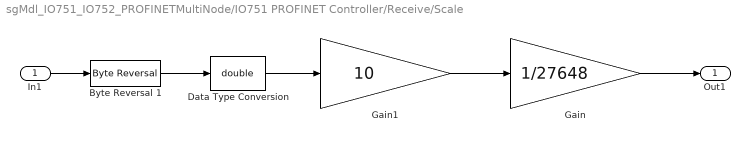
== system sgMdl_IO751_IO752_PROFINETMultiNode/IO751 PROFINET Controller/Receive/Scale ==
  In1 : Inport
  Byte Reversal 1 : slrealtimeutilitieslib/Byte Reversal  numInp=1
  Data Type Conversion : DataTypeConversion  OutDataTypeStr=double  SaturateOnIntegerOverflow=off  RndMeth=Floor
  Gain : Gain  Gain=1/27648
  Gain1 : Gain  Gain=10
  Out1 : Outport
  wires:
  Gain/1 -> Out1/1
  In1/1 -> Byte Reversal 1/1
  Byte Reversal 1/1 -> Data Type Conversion/1
  Data Type Conversion/1 -> Gain1/1
  Gain1/1 -> Gain/1

== system sgMdl_IO751_IO752_PROFINETMultiNode/IO751 PROFINET Controller/Receive/Subsystem ==
  In1 : Inport
  Byte Reversal 4 : slrealtimeutilitieslib/Byte Reversal  numInp=1
  Data Type Conversion1 : DataTypeConversion  OutDataTypeStr=double  SaturateOnIntegerOverflow=off  RndMeth=Floor
  Gain2 : Gain  Gain=1/hex2dec('4000')
  Gain3 : Gain  Gain=8000
  Out1 : Outport
  wires:
  Data Type Conversion1/1 -> Gain3/1
  Byte Reversal 4/1 -> Data Type Conversion1/1
  Gain3/1 -> Gain2/1
  Gain2/1 -> Out1/1
  In1/1 -> Byte Reversal 4/1

== system sgMdl_IO751_IO752_PROFINETMultiNode/IO751 PROFINET Controller/Receive/Subsystem1 ==
  In1 : Inport
  Byte Reversal 1 : slrealtimeutilitieslib/Byte Reversal  numInp=1
  Data Type Conversion2 : DataTypeConversion  OutDataTypeStr=double  SaturateOnIntegerOverflow=off  RndMeth=Floor
  Gain1 : Gain  Gain=1/hex2dec('4000')
  Gain4 : Gain  Gain=8000
  Out1 : Outport
  wires:
  Data Type Conversion2/1 -> Gain4/1
  Byte Reversal 1/1 -> Data Type Conversion2/1
  Gain4/1 -> Gain1/1
  In1/1 -> Byte Reversal 1/1
  Gain1/1 -> Out1/1

== system sgMdl_IO751_IO752_PROFINETMultiNode/IO751 PROFINET Controller/Send/Scale ==
  In1 : Inport
  Byte Reversal 2 : slrealtimeutilitieslib/Byte Reversal  numInp=1
  Data Type Conversion : DataTypeConversion  OutDataTypeStr=int16  SaturateOnIntegerOverflow=off  RndMeth=Floor
  Gain : Gain  Gain=27648
  Gain1 : Gain  Gain=1/10
  Out1 : Outport
  wires:
  Byte Reversal 2/1 -> Out1/1
  Gain/1 -> Gain1/1
  In1/1 -> Gain/1
  Data Type Conversion/1 -> Byte Reversal 2/1
  Gain1/1 -> Data Type Conversion/1

== system sgMdl_IO751_IO752_PROFINETMultiNode/IO751 PROFINET Controller/Send/Scale2 ==
  In1 : Inport
  Byte Reversal 1 : slrealtimeutilitieslib/Byte Reversal  numInp=1
  Data Type Conversion1 : DataTypeConversion  OutDataTypeStr=int16  SaturateOnIntegerOverflow=off  RndMeth=Floor
  Gain2 : Gain  Gain=hex2dec('4000')
  Gain3 : Gain  Gain=1/8000
  Out1 : Outport
  wires:
  Gain2/1 -> Gain3/1
  Byte Reversal 1/1 -> Out1/1
  Gain3/1 -> Data Type Conversion1/1
  Data Type Conversion1/1 -> Byte Reversal 1/1
  In1/1 -> Gain2/1

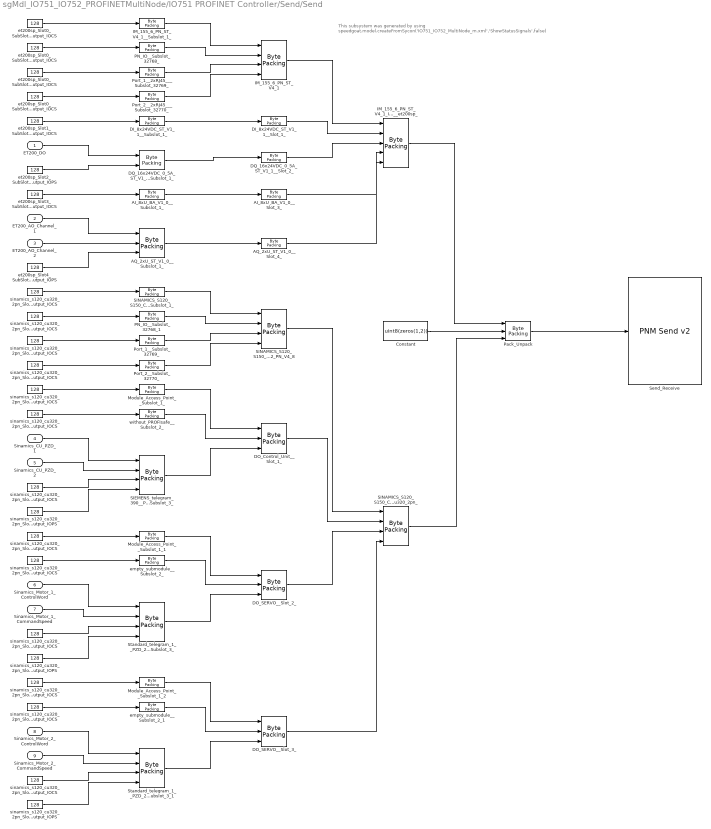
== system sgMdl_IO751_IO752_PROFINETMultiNode/IO751 PROFINET Controller/Send/Send ==
  note: This subsystem was generated by using speedgoat.model.createFromSycon('IO751_IO752_MultiNode_m.xml','ShowStatusSignals',false)
  ET200_DO : Inport  OutDataTypeStr=uint16  PortDimensions=1
  ET200_AO_Channel_1 : Inport  Port=2  OutDataTypeStr=int16  PortDimensions=1
  ET200_AO_Channel_2 : Inport  Port=3  OutDataTypeStr=int16  PortDimensions=1
  Sinamics_CU_PZD_1 : Inport  Port=4  OutDataTypeStr=uint16  PortDimensions=1
  Sinamics_CU_PZD_2 : Inport  Port=5  OutDataTypeStr=uint16  PortDimensions=1
  Sinamics_Motor_1_ControlWord : Inport  Port=6  OutDataTypeStr=uint16  PortDimensions=1
  Sinamics_Motor_1_CommandSpeed : Inport  Port=7  OutDataTypeStr=int16  PortDimensions=1
  Sinamics_Motor_2_ControlWord : Inport  Port=8  OutDataTypeStr=uint16  PortDimensions=1
  Sinamics_Motor_2_CommandSpeed : Inport  Port=9  OutDataTypeStr=int16  PortDimensions=1
  AI_8xU_BA_V1_0__Slot_3_ : slrealtimeutilitieslib/Byte Packing  MaskPackedDataType=uint8  MaskUnpackedDataTypes={'uint8'}  MaskAlignment=1
  AI_8xU_BA_V1_0__Subslot_1_ : slrealtimeutilitieslib/Byte Packing  MaskPackedDataType=uint8  MaskUnpackedDataTypes={'uint8'}  MaskAlignment=1
  AQ_2xU_ST_V1_0__Slot_4_ : slrealtimeutilitieslib/Byte Packing  MaskPackedDataType=uint8  MaskUnpackedDataTypes={'uint8'}  MaskAlignment=1
  AQ_2xU_ST_V1_0__Subslot_1_ : slrealtimeutilitieslib/Byte Packing  MaskPackedDataType=uint8  MaskUnpackedDataTypes={'int16','int16','uint8'}  MaskAlignment=1
  Constant : Constant  Value=uint8(zeros(1,2))
  DI_8x24VDC_ST_V1_1__Slot_1_ : slrealtimeutilitieslib/Byte Packing  MaskPackedDataType=uint8  MaskUnpackedDataTypes={'uint8'}  MaskAlignment=1
  DI_8x24VDC_ST_V1_1__Subslot_1_ : slrealtimeutilitieslib/Byte Packing  MaskPackedDataType=uint8  MaskUnpackedDataTypes={'uint8'}  MaskAlignment=1
  DO_Control_Unit__Slot_1_ : slrealtimeutilitieslib/Byte Packing  MaskPackedDataType=uint8  MaskUnpackedDataTypes={'uint8','uint8','uint8'}  MaskAlignment=1
  DO_SERVO__Slot_2_ : slrealtimeutilitieslib/Byte Packing  MaskPackedDataType=uint8  MaskUnpackedDataTypes={'uint8','uint8','uint8'}  MaskAlignment=1
  DO_SERVO__Slot_3_ : slrealtimeutilitieslib/Byte Packing  MaskPackedDataType=uint8  MaskUnpackedDataTypes={'uint8','uint8','uint8'}  MaskAlignment=1
  DQ_16x24VDC_0_5A_ST_V1_1__Slot_2_ : slrealtimeutilitieslib/Byte Packing  MaskPackedDataType=uint8  MaskUnpackedDataTypes={'uint8'}  MaskAlignment=1
  DQ_16x24VDC_0_5A_ST_V1_1__Subslot_1_ : slrealtimeutilitieslib/Byte Packing  MaskPackedDataType=uint8  MaskUnpackedDataTypes={'uint16','uint8'}  MaskAlignment=1
  IM_155_6_PN_ST_V4_1 : slrealtimeutilitieslib/Byte Packing  MaskPackedDataType=uint8  MaskUnpackedDataTypes={'uint8','uint8','uint8','uint8'}  MaskAlignment=1
  IM_155_6_PN_ST_V4_1_IM_155_6_PN_ST_V4_1__et200sp_ : slrealtimeutilitieslib/Byte Packing  MaskPackedDataType=uint8  MaskUnpackedDataTypes={'uint8','uint8','uint8','uint8','uint8'}  MaskAlignment=1
  IM_155_6_PN_ST_V4_1__Subslot_1_ : slrealtimeutilitieslib/Byte Packing  MaskPackedDataType=uint8  MaskUnpackedDataTypes={'uint8'}  MaskAlignment=1
  Module_Access_Point__Subslot_1_ : slrealtimeutilitieslib/Byte Packing  MaskPackedDataType=uint8  MaskUnpackedDataTypes={'uint8'}  MaskAlignment=1
  Module_Access_Point__Subslot_1_1 : slrealtimeutilitieslib/Byte Packing  MaskPackedDataType=uint8  MaskUnpackedDataTypes={'uint8'}  MaskAlignment=1
  Module_Access_Point__Subslot_1_2 : slrealtimeutilitieslib/Byte Packing  MaskPackedDataType=uint8  MaskUnpackedDataTypes={'uint8'}  MaskAlignment=1
  PN_IO__Subslot_32768_ : slrealtimeutilitieslib/Byte Packing  MaskPackedDataType=uint8  MaskUnpackedDataTypes={'uint8'}  MaskAlignment=1
  PN_IO__Subslot_32768_1 : slrealtimeutilitieslib/Byte Packing  MaskPackedDataType=uint8  MaskUnpackedDataTypes={'uint8'}  MaskAlignment=1
  Pack_Unpack : slrealtimeutilitieslib/Byte Packing  MaskPackedDataType=uint8  MaskUnpackedDataTypes={'uint8','uint8','uint8'}  MaskAlignment=1
  Port_1__2xRJ45___Subslot_32769_ : slrealtimeutilitieslib/Byte Packing  MaskPackedDataType=uint8  MaskUnpackedDataTypes={'uint8'}  MaskAlignment=1
  Port_1__Subslot_32769_ : slrealtimeutilitieslib/Byte Packing  MaskPackedDataType=uint8  MaskUnpackedDataTypes={'uint8'}  MaskAlignment=1
  Port_2__2xRJ45___Subslot_32770_ : slrealtimeutilitieslib/Byte Packing  MaskPackedDataType=uint8  MaskUnpackedDataTypes={'uint8'}  MaskAlignment=1
  Port_2__Subslot_32770_ : slrealtimeutilitieslib/Byte Packing  MaskPackedDataType=uint8  MaskUnpackedDataTypes={'uint8'}  MaskAlignment=1
  SIEMENS_telegram_390__PZD_2_2__Subslot_3_ : slrealtimeutilitieslib/Byte Packing  MaskPackedDataType=uint8  MaskUnpackedDataTypes={'uint16','uint16','uint8','uint8'}  MaskAlignment=1
  SINAMICS_S120_S150_CU320_2_PN_V4_8 : slrealtimeutilitieslib/Byte Packing  MaskPackedDataType=uint8  MaskUnpackedDataTypes={'uint8','uint8','uint8','uint8'}  MaskAlignment=1
  SINAMICS_S120_S150_CU320_2_PN_V4_8_SINAMICS_S120_S150_CU320_2_PN_V4_8__sinamics_s120_cu320_2pn_ : slrealtimeutilitieslib/Byte Packing  MaskPackedDataType=uint8  MaskUnpackedDataTypes={'uint8','uint8','uint8','uint8'}  MaskAlignment=1
  SINAMICS_S120_S150_CU320_2_PN_V4_8__Subslot_1_ : slrealtimeutilitieslib/Byte Packing  MaskPackedDataType=uint8  MaskUnpackedDataTypes={'uint8'}  MaskAlignment=1
  Send_Receive : speedgoatlib_IO751/PNM Send v2   id=1  portType=1 port with n element vector of type UINT8  inputOutput=44  sampleTime=Ts
      settings: SourceProductName=IO751 PROFINET Controller
  Standard_telegram_1__PZD_2_2__Subslot_3_ : slrealtimeutilitieslib/Byte Packing  MaskPackedDataType=uint8  MaskUnpackedDataTypes={'uint16','int16','uint8','uint8'}  MaskAlignment=1
  Standard_telegram_1__PZD_2_2__Subslot_3_1 : slrealtimeutilitieslib/Byte Packing  MaskPackedDataType=uint8  MaskUnpackedDataTypes={'uint16','int16','uint8','uint8'}  MaskAlignment=1
  empty_submodule__Subslot_2_ : slrealtimeutilitieslib/Byte Packing  MaskPackedDataType=uint8  MaskUnpackedDataTypes={'uint8'}  MaskAlignment=1
  empty_submodule__Subslot_2_1 : slrealtimeutilitieslib/Byte Packing  MaskPackedDataType=uint8  MaskUnpackedDataTypes={'uint8'}  MaskAlignment=1
  et200sp_Slot0_SubSlot1_Output_IOCS : Constant  Value=128  OutDataTypeStr=uint8
  et200sp_Slot0_SubSlot32768_Output_IOCS : Constant  Value=128  OutDataTypeStr=uint8
  et200sp_Slot0_SubSlot32769_Output_IOCS : Constant  Value=128  OutDataTypeStr=uint8
  et200sp_Slot0_SubSlot32770_Output_IOCS : Constant  Value=128  OutDataTypeStr=uint8
  et200sp_Slot1_SubSlot1_Output_IOCS : Constant  Value=128  OutDataTypeStr=uint8
  et200sp_Slot2_SubSlot1_Output_IOPS : Constant  Value=128  OutDataTypeStr=uint8
  et200sp_Slot3_SubSlot1_Output_IOCS : Constant  Value=128  OutDataTypeStr=uint8
  et200sp_Slot4_SubSlot1_Output_IOPS : Constant  Value=128  OutDataTypeStr=uint8
  sinamics_s120_cu320_2pn_Slot0_SubSlot1_Output_IOCS : Constant  Value=128  OutDataTypeStr=uint8
  sinamics_s120_cu320_2pn_Slot0_SubSlot32768_Output_IOCS : Constant  Value=128  OutDataTypeStr=uint8
  sinamics_s120_cu320_2pn_Slot0_SubSlot32769_Output_IOCS : Constant  Value=128  OutDataTypeStr=uint8
  sinamics_s120_cu320_2pn_Slot0_SubSlot32770_Output_IOCS : Constant  Value=128  OutDataTypeStr=uint8
  sinamics_s120_cu320_2pn_Slot1_SubSlot1_Output_IOCS : Constant  Value=128  OutDataTypeStr=uint8
  sinamics_s120_cu320_2pn_Slot1_SubSlot2_Output_IOCS : Constant  Value=128  OutDataTypeStr=uint8
  sinamics_s120_cu320_2pn_Slot1_SubSlot3_Output_IOCS : Constant  Value=128  OutDataTypeStr=uint8
  sinamics_s120_cu320_2pn_Slot1_SubSlot3_Output_IOPS : Constant  Value=128  OutDataTypeStr=uint8
  sinamics_s120_cu320_2pn_Slot2_SubSlot1_Output_IOCS : Constant  Value=128  OutDataTypeStr=uint8
  sinamics_s120_cu320_2pn_Slot2_SubSlot2_Output_IOCS : Constant  Value=128  OutDataTypeStr=uint8
  sinamics_s120_cu320_2pn_Slot2_SubSlot3_Output_IOCS : Constant  Value=128  OutDataTypeStr=uint8
  sinamics_s120_cu320_2pn_Slot2_SubSlot3_Output_IOPS : Constant  Value=128  OutDataTypeStr=uint8
  sinamics_s120_cu320_2pn_Slot3_SubSlot1_Output_IOCS : Constant  Value=128  OutDataTypeStr=uint8
  sinamics_s120_cu320_2pn_Slot3_SubSlot2_Output_IOCS : Constant  Value=128  OutDataTypeStr=uint8
  sinamics_s120_cu320_2pn_Slot3_SubSlot3_Output_IOCS : Constant  Value=128  OutDataTypeStr=uint8
  sinamics_s120_cu320_2pn_Slot3_SubSlot3_Output_IOPS : Constant  Value=128  OutDataTypeStr=uint8
  without_PROFIsafe__Subslot_2_ : slrealtimeutilitieslib/Byte Packing  MaskPackedDataType=uint8  MaskUnpackedDataTypes={'uint8'}  MaskAlignment=1
  wires:
  et200sp_Slot0_SubSlot1_Output_IOCS/1 -> IM_155_6_PN_ST_V4_1__Subslot_1_/1
  et200sp_Slot0_SubSlot32768_Output_IOCS/1 -> PN_IO__Subslot_32768_/1
  et200sp_Slot0_SubSlot32769_Output_IOCS/1 -> Port_1__2xRJ45___Subslot_32769_/1
  et200sp_Slot0_SubSlot32770_Output_IOCS/1 -> Port_2__2xRJ45___Subslot_32770_/1
  IM_155_6_PN_ST_V4_1__Subslot_1_/1 -> IM_155_6_PN_ST_V4_1/1
  PN_IO__Subslot_32768_/1 -> IM_155_6_PN_ST_V4_1/2
  Port_1__2xRJ45___Subslot_32769_/1 -> IM_155_6_PN_ST_V4_1/3
  Port_2__2xRJ45___Subslot_32770_/1 -> IM_155_6_PN_ST_V4_1/4
  et200sp_Slot1_SubSlot1_Output_IOCS/1 -> DI_8x24VDC_ST_V1_1__Subslot_1_/1
  DI_8x24VDC_ST_V1_1__Subslot_1_/1 -> DI_8x24VDC_ST_V1_1__Slot_1_/1
  ET200_DO/1 -> DQ_16x24VDC_0_5A_ST_V1_1__Subslot_1_/1
  et200sp_Slot2_SubSlot1_Output_IOPS/1 -> DQ_16x24VDC_0_5A_ST_V1_1__Subslot_1_/2
  DQ_16x24VDC_0_5A_ST_V1_1__Subslot_1_/1 -> DQ_16x24VDC_0_5A_ST_V1_1__Slot_2_/1
  et200sp_Slot3_SubSlot1_Output_IOCS/1 -> AI_8xU_BA_V1_0__Subslot_1_/1
  AI_8xU_BA_V1_0__Subslot_1_/1 -> AI_8xU_BA_V1_0__Slot_3_/1
  ET200_AO_Channel_1/1 -> AQ_2xU_ST_V1_0__Subslot_1_/1
  ET200_AO_Channel_2/1 -> AQ_2xU_ST_V1_0__Subslot_1_/2
  et200sp_Slot4_SubSlot1_Output_IOPS/1 -> AQ_2xU_ST_V1_0__Subslot_1_/3
  AQ_2xU_ST_V1_0__Subslot_1_/1 -> AQ_2xU_ST_V1_0__Slot_4_/1
  IM_155_6_PN_ST_V4_1/1 -> IM_155_6_PN_ST_V4_1_IM_155_6_PN_ST_V4_1__et200sp_/1
  DI_8x24VDC_ST_V1_1__Slot_1_/1 -> IM_155_6_PN_ST_V4_1_IM_155_6_PN_ST_V4_1__et200sp_/2
  DQ_16x24VDC_0_5A_ST_V1_1__Slot_2_/1 -> IM_155_6_PN_ST_V4_1_IM_155_6_PN_ST_V4_1__et200sp_/3
  AI_8xU_BA_V1_0__Slot_3_/1 -> IM_155_6_PN_ST_V4_1_IM_155_6_PN_ST_V4_1__et200sp_/4
  AQ_2xU_ST_V1_0__Slot_4_/1 -> IM_155_6_PN_ST_V4_1_IM_155_6_PN_ST_V4_1__et200sp_/5
  sinamics_s120_cu320_2pn_Slot0_SubSlot1_Output_IOCS/1 -> SINAMICS_S120_S150_CU320_2_PN_V4_8__Subslot_1_/1
  sinamics_s120_cu320_2pn_Slot0_SubSlot32768_Output_IOCS/1 -> PN_IO__Subslot_32768_1/1
  sinamics_s120_cu320_2pn_Slot0_SubSlot32769_Output_IOCS/1 -> Port_1__Subslot_32769_/1
  sinamics_s120_cu320_2pn_Slot0_SubSlot32770_Output_IOCS/1 -> Port_2__Subslot_32770_/1
  SINAMICS_S120_S150_CU320_2_PN_V4_8__Subslot_1_/1 -> SINAMICS_S120_S150_CU320_2_PN_V4_8/1
  PN_IO__Subslot_32768_1/1 -> SINAMICS_S120_S150_CU320_2_PN_V4_8/2
  Port_1__Subslot_32769_/1 -> SINAMICS_S120_S150_CU320_2_PN_V4_8/3
  Port_2__Subslot_32770_/1 -> SINAMICS_S120_S150_CU320_2_PN_V4_8/4
  sinamics_s120_cu320_2pn_Slot1_SubSlot1_Output_IOCS/1 -> Module_Access_Point__Subslot_1_/1
  sinamics_s120_cu320_2pn_Slot1_SubSlot2_Output_IOCS/1 -> without_PROFIsafe__Subslot_2_/1
  Sinamics_CU_PZD_1/1 -> SIEMENS_telegram_390__PZD_2_2__Subslot_3_/1
  Sinamics_CU_PZD_2/1 -> SIEMENS_telegram_390__PZD_2_2__Subslot_3_/2
  sinamics_s120_cu320_2pn_Slot1_SubSlot3_Output_IOCS/1 -> SIEMENS_telegram_390__PZD_2_2__Subslot_3_/3
  sinamics_s120_cu320_2pn_Slot1_SubSlot3_Output_IOPS/1 -> SIEMENS_telegram_390__PZD_2_2__Subslot_3_/4
  Module_Access_Point__Subslot_1_/1 -> DO_Control_Unit__Slot_1_/1
  without_PROFIsafe__Subslot_2_/1 -> DO_Control_Unit__Slot_1_/2
  SIEMENS_telegram_390__PZD_2_2__Subslot_3_/1 -> DO_Control_Unit__Slot_1_/3
  sinamics_s120_cu320_2pn_Slot2_SubSlot1_Output_IOCS/1 -> Module_Access_Point__Subslot_1_1/1
  sinamics_s120_cu320_2pn_Slot2_SubSlot2_Output_IOCS/1 -> empty_submodule__Subslot_2_/1
  Sinamics_Motor_1_ControlWord/1 -> Standard_telegram_1__PZD_2_2__Subslot_3_/1
  Sinamics_Motor_1_CommandSpeed/1 -> Standard_telegram_1__PZD_2_2__Subslot_3_/2
  sinamics_s120_cu320_2pn_Slot2_SubSlot3_Output_IOCS/1 -> Standard_telegram_1__PZD_2_2__Subslot_3_/3
  sinamics_s120_cu320_2pn_Slot2_SubSlot3_Output_IOPS/1 -> Standard_telegram_1__PZD_2_2__Subslot_3_/4
  Module_Access_Point__Subslot_1_1/1 -> DO_SERVO__Slot_2_/1
  empty_submodule__Subslot_2_/1 -> DO_SERVO__Slot_2_/2
  Standard_telegram_1__PZD_2_2__Subslot_3_/1 -> DO_SERVO__Slot_2_/3
  sinamics_s120_cu320_2pn_Slot3_SubSlot1_Output_IOCS/1 -> Module_Access_Point__Subslot_1_2/1
  sinamics_s120_cu320_2pn_Slot3_SubSlot2_Output_IOCS/1 -> empty_submodule__Subslot_2_1/1
  Sinamics_Motor_2_ControlWord/1 -> Standard_telegram_1__PZD_2_2__Subslot_3_1/1
  Sinamics_Motor_2_CommandSpeed/1 -> Standard_telegram_1__PZD_2_2__Subslot_3_1/2
  sinamics_s120_cu320_2pn_Slot3_SubSlot3_Output_IOCS/1 -> Standard_telegram_1__PZD_2_2__Subslot_3_1/3
  sinamics_s120_cu320_2pn_Slot3_SubSlot3_Output_IOPS/1 -> Standard_telegram_1__PZD_2_2__Subslot_3_1/4
  Module_Access_Point__Subslot_1_2/1 -> DO_SERVO__Slot_3_/1
  empty_submodule__Subslot_2_1/1 -> DO_SERVO__Slot_3_/2
  Standard_telegram_1__PZD_2_2__Subslot_3_1/1 -> DO_SERVO__Slot_3_/3
  SINAMICS_S120_S150_CU320_2_PN_V4_8/1 -> SINAMICS_S120_S150_CU320_2_PN_V4_8_SINAMICS_S120_S150_CU320_2_PN_V4_8__sinamics_s120_cu320_2pn_/1
  DO_Control_Unit__Slot_1_/1 -> SINAMICS_S120_S150_CU320_2_PN_V4_8_SINAMICS_S120_S150_CU320_2_PN_V4_8__sinamics_s120_cu320_2pn_/2
  DO_SERVO__Slot_2_/1 -> SINAMICS_S120_S150_CU320_2_PN_V4_8_SINAMICS_S120_S150_CU320_2_PN_V4_8__sinamics_s120_cu320_2pn_/3
  DO_SERVO__Slot_3_/1 -> SINAMICS_S120_S150_CU320_2_PN_V4_8_SINAMICS_S120_S150_CU320_2_PN_V4_8__sinamics_s120_cu320_2pn_/4
  IM_155_6_PN_ST_V4_1_IM_155_6_PN_ST_V4_1__et200sp_/1 -> Pack_Unpack/1
  Pack_Unpack/1 -> Send_Receive/1
  SINAMICS_S120_S150_CU320_2_PN_V4_8_SINAMICS_S120_S150_CU320_2_PN_V4_8__sinamics_s120_cu320_2pn_/1 -> Pack_Unpack/3
  Constant/1 -> Pack_Unpack/2

== system sgMdl_IO751_IO752_PROFINETMultiNode/IO752-32 PROFINET Device Simulation/Device 1 ET200SP/Scale ==
  In1 : Inport
  Byte Reversal : slrealtimeutilitieslib/Byte Reversal  numInp=1
  Data Type Conversion : DataTypeConversion  OutDataTypeStr=double  SaturateOnIntegerOverflow=off  RndMeth=Floor
  Gain : Gain  Gain=1/27648
  Gain1 : Gain  Gain=10
  Out1 : Outport
  wires:
  Gain/1 -> Out1/1
  In1/1 -> Byte Reversal/1
  Byte Reversal/1 -> Data Type Conversion/1
  Data Type Conversion/1 -> Gain1/1
  Gain1/1 -> Gain/1

== system sgMdl_IO751_IO752_PROFINETMultiNode/IO752-32 PROFINET Device Simulation/Device 1 ET200SP/Scale1 ==
  In1 : Inport
  Byte Reversal 2 : slrealtimeutilitieslib/Byte Reversal  numInp=1
  Data Type Conversion : DataTypeConversion  OutDataTypeStr=int16  SaturateOnIntegerOverflow=off  RndMeth=Floor
  Gain : Gain  Gain=27648
  Gain1 : Gain  Gain=1/10
  Out1 : Outport
  wires:
  Byte Reversal 2/1 -> Out1/1
  Gain/1 -> Gain1/1
  In1/1 -> Gain/1
  Data Type Conversion/1 -> Byte Reversal 2/1
  Gain1/1 -> Data Type Conversion/1

== system sgMdl_IO751_IO752_PROFINETMultiNode/IO752-32 PROFINET Device Simulation/Device 2 SINAMICS/PT1-Delay ==
  u : Inport
  Sum : Sum  Inputs=|++  OutDataTypeStr=double  AccumDataTypeStr=double
  "feedback_gain " : Gain  Gain=-10.0  OutDataTypeStr=double
  input_gain : Gain  Gain=10.0
  integrator : DiscreteIntegrator  SampleTime=Ts  OutDataTypeStr=double  ICPrevOutput=DiscIntNeverNeededParam  ICPrevScaledInput=DiscIntNeverNeededParam
  y : Outport  VectorParamsAs1DForOutWhenUnconnected=off
  wires:
  u/1 -> input_gain/1
  integrator/1 -> y/1, "feedback_gain "/1
  Sum/1 -> integrator/1
  "feedback_gain "/1 -> Sum/2
  input_gain/1 -> Sum/1

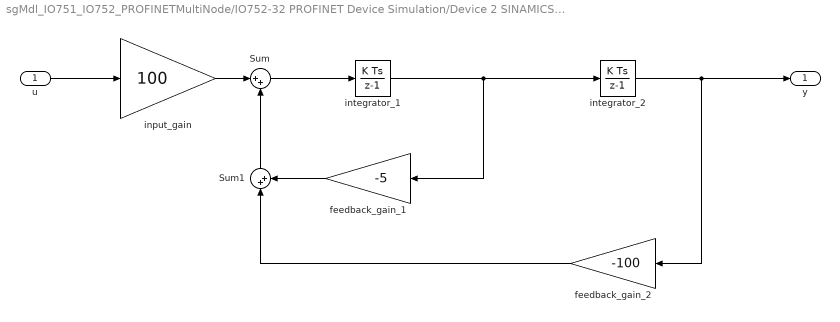
== system sgMdl_IO751_IO752_PROFINETMultiNode/IO752-32 PROFINET Device Simulation/Device 2 SINAMICS/PT2-Delay ==
  u : Inport
  Sum : Sum  Inputs=|++
  Sum1 : Sum  Inputs=|++
  feedback_gain_1 : Gain  Gain=-5
  feedback_gain_2 : Gain  Gain=-100
  input_gain : Gain  Gain=100
  integrator_1 : DiscreteIntegrator  gainval=2  SampleTime=0.001  ICPrevOutput=DiscIntNeverNeededParam  ICPrevScaledInput=DiscIntNeverNeededParam
  integrator_2 : DiscreteIntegrator  gainval=2  SampleTime=0.001  ICPrevOutput=DiscIntNeverNeededParam  ICPrevScaledInput=DiscIntNeverNeededParam
  y : Outport  VectorParamsAs1DForOutWhenUnconnected=off
  wires:
  feedback_gain_2/1 -> Sum1/1
  integrator_2/1 -> y/1, feedback_gain_2/1
  feedback_gain_1/1 -> Sum1/2
  input_gain/1 -> Sum/1
  Sum/1 -> integrator_1/1
  integrator_1/1 -> integrator_2/1, feedback_gain_1/1
  Sum1/1 -> Sum/2
  u/1 -> input_gain/1

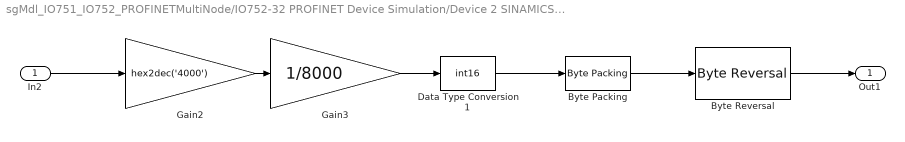
== system sgMdl_IO751_IO752_PROFINETMultiNode/IO752-32 PROFINET Device Simulation/Device 2 SINAMICS/Scale1 ==
  In2 : Inport  PortDimensions=1
  Byte Packing : slrealtimeutilitieslib/Byte Packing  MaskPackedDataType=uint16  MaskUnpackedDataTypes={'int16'}  MaskAlignment=1
  Byte Reversal : slrealtimeutilitieslib/Byte Reversal  numInp=1
  Data Type Conversion1 : DataTypeConversion  OutDataTypeStr=int16  SaturateOnIntegerOverflow=off  RndMeth=Floor
  Gain2 : Gain  Gain=hex2dec('4000')
  Gain3 : Gain  Gain=1/8000
  Out1 : Outport
  wires:
  Gain2/1 -> Gain3/1
  Gain3/1 -> Data Type Conversion1/1
  Byte Reversal/1 -> Out1/1
  Data Type Conversion1/1 -> Byte Packing/1
  Byte Packing/1 -> Byte Reversal/1
  In2/1 -> Gain2/1

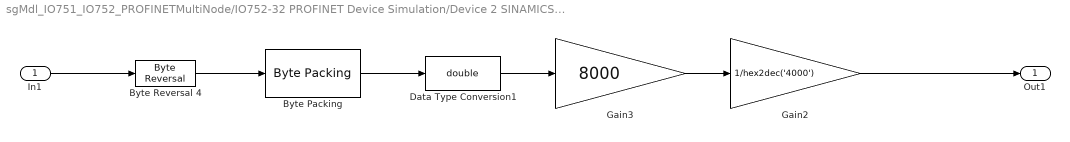
== system sgMdl_IO751_IO752_PROFINETMultiNode/IO752-32 PROFINET Device Simulation/Device 2 SINAMICS/Scale2 ==
  In1 : Inport
  Byte Packing : slrealtimeutilitieslib/Byte Packing  MaskPackedDataType=int16  MaskUnpackedDataTypes={'uint16'}  MaskAlignment=1
  Byte Reversal 4 : slrealtimeutilitieslib/Byte Reversal  numInp=1
  Data Type Conversion1 : DataTypeConversion  OutDataTypeStr=double  SaturateOnIntegerOverflow=off  RndMeth=Floor
  Gain2 : Gain  Gain=1/hex2dec('4000')
  Gain3 : Gain  Gain=8000
  Out1 : Outport
  wires:
  Data Type Conversion1/1 -> Gain3/1
  Byte Reversal 4/1 -> Byte Packing/1
  Gain3/1 -> Gain2/1
  Gain2/1 -> Out1/1
  In1/1 -> Byte Reversal 4/1
  Byte Packing/1 -> Data Type Conversion1/1
